simulink model "RL_train_simulation"  (R2024a)
settings: Solver=VariableStepAuto  StartTime=0.0  StopTime=10.0  RelTol=1e-3
libraries: Solver_SF x1, rllib x1
settings Model: Creator=14708  LastModifiedBy=14708

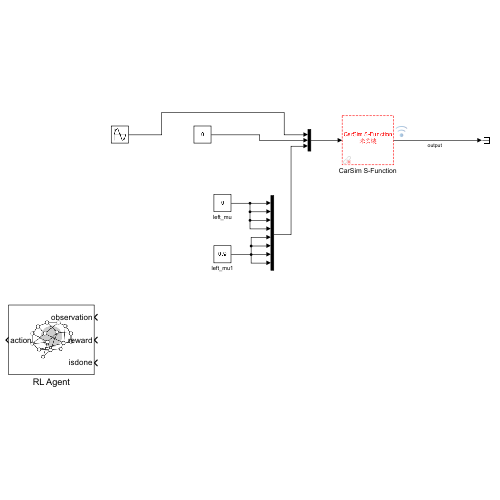
[thumbnail: Simulink's stored preview of the top-level diagram]
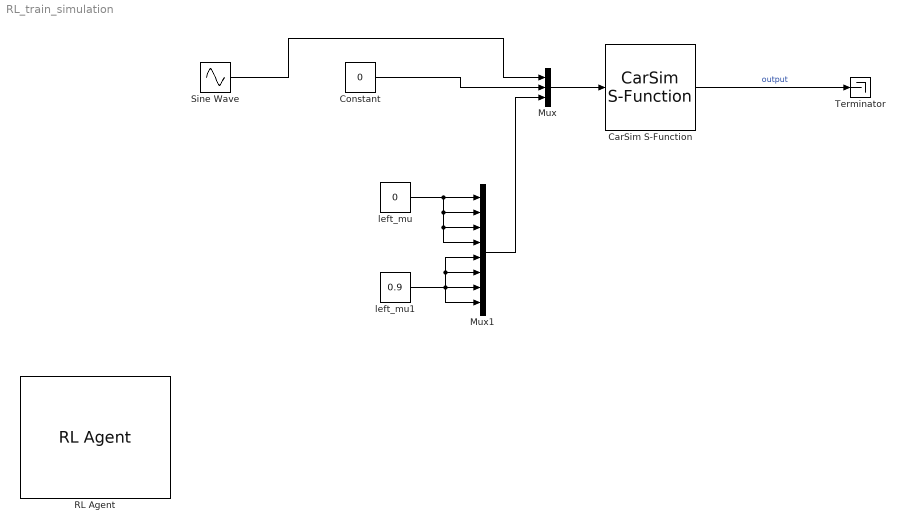
== system RL_train_simulation ==
  CarSim S-Function : Solver_SF/CarSim S-Function  Priority=1  SIMFILE=simfile.sim  Run_RTs=off  vs_state_ind=Run  StopMode_ind=Vehicle Model
  Constant : Constant  Value=0
  Mux : Mux  Inputs=3
  Mux1 : Mux  Inputs=8
  RL Agent : rllib/RL Agent  Agent=agent  ExternalActionAsInput=off  ProvideLastAction=off  ProvideCumRwd=off  TreatAsDirectFeedthrough=on  UseStrictObservationDataTypes=off
  Sine Wave : Sin  Amplitude=500  SampleTime=0
  Terminator : Terminator
  left_mu : Constant  Value=0
  left_mu1 : Constant  Value=0.9
  wires:
  CarSim S-Function/1 -> Terminator/1  "output"
  left_mu/1 -> Mux1/4, Mux1/3, Mux1/2, Mux1/1
  left_mu1/1 -> Mux1/5, Mux1/6, Mux1/8, Mux1/7
  Constant/1 -> Mux/2
  Mux1/1 -> Mux/3
  Mux/1 -> CarSim S-Function/1
  Sine Wave/1 -> Mux/1
